simulink library "wheel_chassis"  (R2024b)
settings: Solver=VariableStepAuto  StartTime=0.0  StopTime=10.0  RelTol=1e-3
undefined symbols (not defined in the file or in its folder): Ke, Kt, n, Ra, Rw, Ts, Vmax
libraries: motor_jgb37 x1, simulink x1
settings Model: Creator=Austinchao  LastModifiedBy=Austinchao

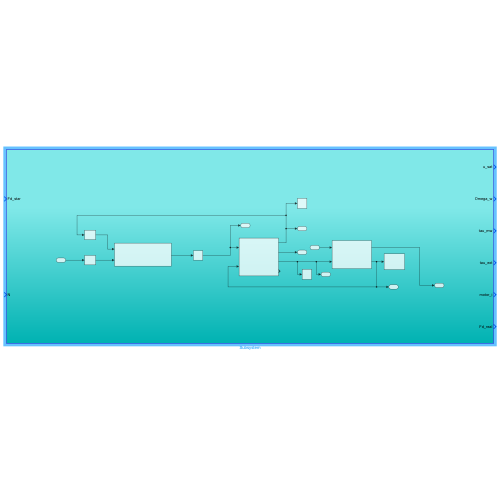
[thumbnail: Simulink's stored preview of the top-level diagram]
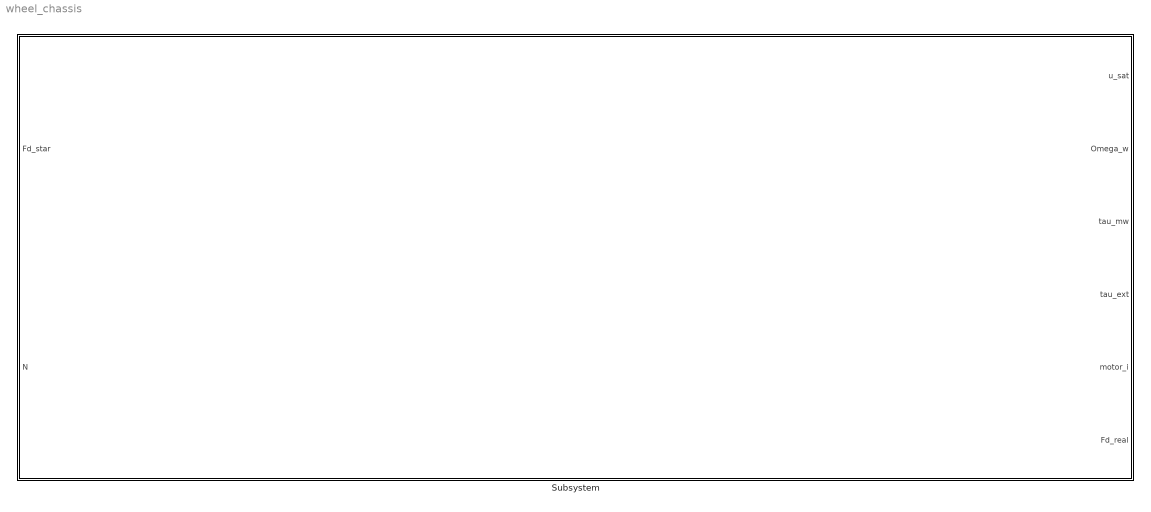
== system wheel_chassis ==
  Subsystem : Subsystem

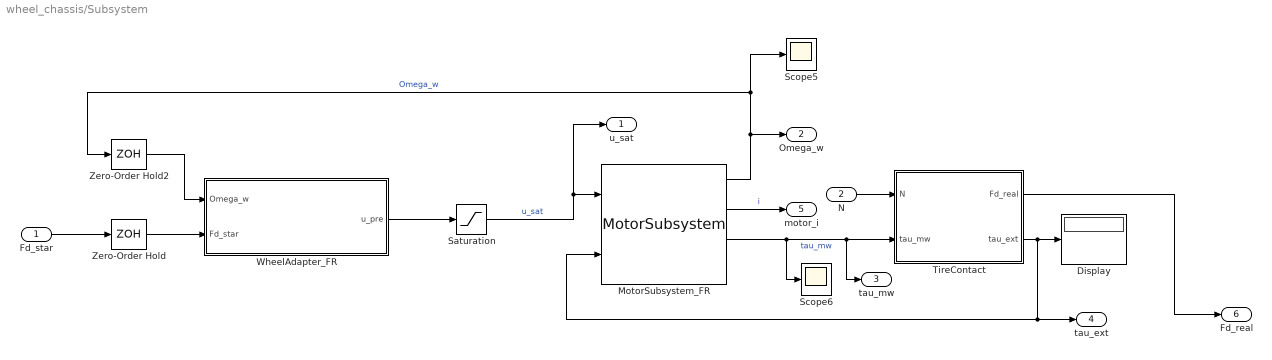
== system wheel_chassis/Subsystem ==
  Fd_star : Inport
  N : Inport  Port=2
  Display : Display
  MotorSubsystem_FR : motor_jgb37/MotorSubsystem  Ra=Ra  Kt=Kt  Ke=Ke  n=n  Rw=Rw  Jm=1*10^-5  Jw=1*10^-4  Bm=3.95*10^-7  tau_c=0  dz=0  Ts=Ts  Bw=0
      settings: SourceProductName=My Library
  Saturation : Saturate  UpperLimit=Vmax  LowerLimit=0
  Scope5 : Scope
  Scope6 : Scope
  TireContact : Subsystem  mask{mu=0.5}
      mask prompts: mu "μ (friction_coefficient)"
  WheelAdapter_FR : MATLAB Function  TreatAsAtomicUnit=on  mask{Rw=Rw, n=n, Ra=Ra, Kt=Kt, Ke=Ke, Ts=Ts, Kp=0}
      mask prompts: Rw "Rw: Wheel radius (m)"; n "n: Gear ratio"; Ra "Ra: Armature resistance (Ohm)"; Kt "Kt: Torque constant (Nm/A)"; Ke "Ke: Back-EMF constant (V/(rad/s))"
  Zero-Order Hold : ZeroOrderHold  SampleTime=Ts
  Zero-Order Hold2 : ZeroOrderHold  SampleTime=Ts
  u_sat : Outport
  Omega_w : Outport  Port=2
  tau_mw : Outport  Port=3
  tau_ext : Outport  Port=4
  motor_i : Outport  Port=5
  Fd_real : Outport  Port=6
  wires:
  MotorSubsystem_FR/1 -> Omega_w/1, Scope5/1, Zero-Order Hold2/1  "Omega_w"
  MotorSubsystem_FR/3 -> Scope6/1, tau_mw/1, TireContact/2(tau_mw)  "tau_mw"
  Zero-Order Hold2/1 -> WheelAdapter_FR/1(Omega_w)
  WheelAdapter_FR/1(u_pre) -> Saturation/1
  Zero-Order Hold/1 -> WheelAdapter_FR/2(Fd_star)
  TireContact/2(tau_ext) -> Display/1, MotorSubsystem_FR/2, tau_ext/1
  Saturation/1 -> u_sat/1, MotorSubsystem_FR/1  "u_sat"
  Fd_star/1 -> Zero-Order Hold/1
  TireContact/1(Fd_real) -> Fd_real/1
  N/1 -> TireContact/1(N)
  MotorSubsystem_FR/2 -> motor_i/1  "i"

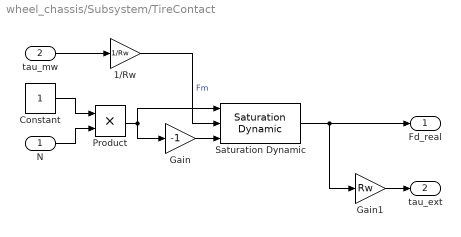
== system wheel_chassis/Subsystem/TireContact ==
  N : Inport
  tau_mw : Inport  Port=2
  1/Rw : Gain  Gain=1/Rw
  Constant : Constant
  Gain : Gain  Gain=-1
  Gain1 : Gain  Gain=Rw
  Product : Product
  Saturation Dynamic : simulink/Discontinuities/Saturation Dynamic  OutMin=[]  OutMax=[]  OutDataTypeStr=Inherit: Same as second input  OutDataType=fixdt(1, 16)  OutScaling=2^-10  DoSatur=off
  Fd_real : Outport
  tau_ext : Outport  Port=2
  wires:
  tau_mw/1 -> 1/Rw/1
  Constant/1 -> Product/1
  N/1 -> Product/2
  Product/1 -> Gain/1, Saturation Dynamic/1
  Gain/1 -> Saturation Dynamic/3
  1/Rw/1 -> Saturation Dynamic/2  "Fm"
  Saturation Dynamic/1 -> Gain1/1, Fd_real/1
  Gain1/1 -> tau_ext/1

== matlab function wheel_chassis/Subsystem/WheelAdapter_FR ==
  data: Omega_w input; Fd_star input; Rw parameter; n parameter; Ra parameter; Kt parameter; Ke parameter; u_pre output
function u_pre  = WheelAdapter(Omega_w,Fd_star, Rw, n, Ra, Kt, Ke)
%persistent I; if isempty(I), I = 0; end
% Fd_star : 期望輪力 (來自 ForceMixer)
% Fd_meas : 實際輸出輪力 (來自 MotorSubsystem)
% Omega_w : 輪速 (來自 MotorSubsystem)

% Mask 參數（之後會在 Mask 裡設定）
% Rw  : 輪半徑 [m]
% n   : 減速比
% Ra  : 電阻 [Ohm]
% Kt  : 轉矩常數 [Nm/A]
% Ke  : 反電動勢常數 [V/(rad/s)]

% 期望輪扭矩
tau_w_star = Rw * Fd_star;

% 前饋電壓
u_ff = (Ra/(Kt*n)) * tau_w_star + (Ke*n) * Omega_w;

% 誤差與比例動作
e     = Fd_star - Fd_meas;
u_pre = u_ff ;

end
